simulink model "Copy_of_neural_network_training"  (R2019a)
settings: Solver=FixedStepAuto  StartTime=0.0  StopTime=500  FixedStep=Ts  RelTol=1e-3  EnableMultiTasking=on
values from neighbouring files (symbols this model uses):
  f1_off = 0    [vreflex.m]
  f2_off = 0    [vreflex.m]
  f3_off = 0    [vreflex.m]
  f4_off = 0    [vreflex.m]
  f5_off = 0    [vreflex.m]
  f6_off = 0    [vreflex.m]
  trial = str2double(get(handles.tryno,'String'))    [vreflex.m]
  Ts = 0.0005    [vreflex.m]
  weight = evalin('base','weight')    [vreflex.m]
undefined symbols (not defined in the file or in its folder): filt_den, filt_num, Pull, up
libraries: dspsigops x9, speedgoatlib_IO183 x6, slrtlib x5, dspswit3 x1, dspstat3 x1, simulink x1
settings Model: Creator=vnalam  LastModifiedBy=vnalam
settings DataIOCC: LimitDataPoints=on  SaveFormat=StructureWithTime  ReturnWorkspaceOutputs=off
settings OptimizationCC: BlockReduction=off  OptimizeBlockIOStorage=off  BufferReuse=off  GlobalBufferReuse=off  ExpressionFolding=off  LocalBlockOutputs=off  LifeSpan=inf  OptimizeDataStoreBuffers=off  BusAssignmentInplaceUpdate=off
settings DebuggingCC: AllowSymbolicDim=off  SFUnexpectedBacktrackingDiag=warning  SFNoUnconditionalDefaultTransitionDiag=warning  SFExecutionAtInitializationDiag=none  ArithmeticOperatorsInVariantConditions=warning
settings HardwareCC: ProdBitPerPointer=32  ProdBitPerSizeT=32  ProdBitPerPtrDiffT=32  ProdLargestAtomicFloat=None  ProdWordSize=32  ProdLongLongMode=on  ProdHWDeviceType=Generic->32-bit x86 compatible
settings ModelReferenceCC: PropagateSignalLabelsOutOfModel=off
settings SFSimCC: SimUseLocalCustomCode=off
settings RTWCC: SystemTargetFile=slrt.tlc  TLCOptions=-axPCModelStackSizeKB=512  TemplateMakefile=slrt_default_tmf  Description=Simulink Real-Time  RTWUseLocalCustomCode=off  CodeExecutionProfiling=on  RTWCompilerOptimization=on
settings CodeAppCC: StateflowObjectComments=on
settings SimulinkRealTimeCC: PreserveStateflowLocalDataDimensions=off  xPCisDownloadable=off
settings ConfigComp: CovMetricSettings=dw  CovHtmlReporting=on  CovSaveCumulativeToWorkspaceVar=on  CovSaveSingleToWorkspaceVar=on  CovExternalEMLEnable=off

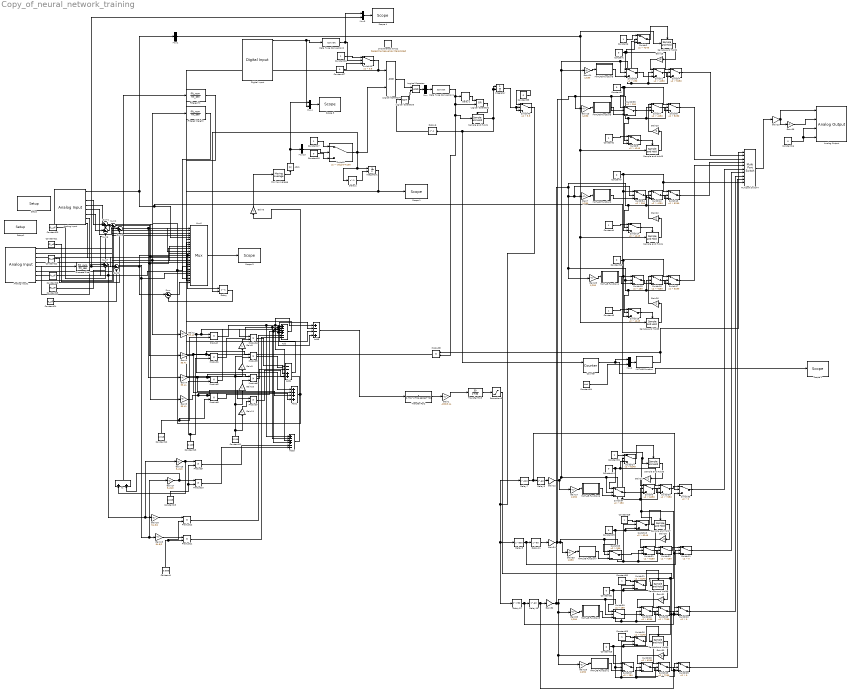
== system Copy_of_neural_network_training ==
  Abs1 : Abs
  Add : Sum  Inputs=+--+--
  Add1 : Sum  Inputs=--++
  Add2 : Sum  Inputs=++++
  Add3 : Sum  Inputs=+--+--
  Add5 : Sum  Inputs=+--+
  Analog Input : speedgoatlib_IO183/Analog Input  Priority=0  parModuleId=1  parSampTime=Ts  parPciSlot=-1  parAdChannelLow=1  parAdChannelHigh=8
      settings: SourceProductName=Simulink Real-Time: Speedgoat Library
  Analog Input1 : speedgoatlib_IO183/Analog Input  Priority=0  parModuleId=2  parSampTime=Ts  parPciSlot=-1  parAdChannelLow=1  parAdChannelHigh=8
      settings: SourceProductName=Simulink Real-Time: Speedgoat Library
  Analog Output : speedgoatlib_IO183/Analog Output  parModuleId=1  parSampTime=-1  parDaSimult=on  parPciSlot=-1  parDaChannels=[1 2 3 4]  parDaInit=[0 0 0 0]  parDaReset=[0 0 0 0]
      settings: SourceProductName=Simulink Real-Time: Speedgoat Library
  Constant{,3,7,10,14..16,18,27,29,31,35} (12 alike) : Constant  Value=0  SampleTime=Ts
  Constant1 : Constant  Value=0.095  SampleTime=-1
  Constant11 : Constant  Value=0.110  SampleTime=-1
  Constant12 : Constant  Value=0.315  SampleTime=-1
  Constant13 : Constant  Value=0.105  SampleTime=-1
  Constant{2,4..6,17,26,28,30,32..33} (10 alike) : Constant  SampleTime=Ts
  Constant19 : Constant  Value=0.025  SampleTime=-1
  Constant20 : Constant  Value=f1_off  SampleTime=Ts
  Constant21 : Constant  Value=f2_off  SampleTime=Ts
  Constant22 : Constant  Value=f3_off  SampleTime=Ts
  Constant23 : Constant  Value=f4_off  SampleTime=Ts
  Constant24 : Constant  Value=f6_off  SampleTime=Ts
  Constant25 : Constant  Value=f5_off  SampleTime=Ts
  Constant34 : Constant  Value=trial  SampleTime=Ts
  Counter : dspswit3/Counter  Direction=Up  CountEvent=Rising edge  CounterSize=User defined  MaxCount=255  InitialCount=0  Output=Count and Hit  HitValue=32  ResetInput=on  SamplesPerFrame=1  Ts=1  CntDtype=double  HitDtype=Boolean
  Data Type Conversion1 : DataTypeConversion
  Data Type Conversion2 : DataTypeConversion
  Delay : Delay  DelayLength=1  ShowEnablePort=on
      settings: InputPortMap=u0,e6
  Delay1 : Delay  DelayLength=12000  InitialCondition=0  SampleTime=Ts
  Delay11 : Delay  DelayLength=60  InitialCondition=0  SampleTime=Ts
  Delay12 : Delay  DelayLength=780  InitialCondition=0  SampleTime=Ts
  Delay13 : Delay  DelayLength=60  InitialCondition=0  SampleTime=Ts
  Delay2 : Delay  DelayLength=1  InitialCondition=0  SampleTime=Ts
  Delay6 : Delay  DelayLength=1  InitialCondition=0  SampleTime=Ts
  Delay7 : Delay  DelayLength=220  InitialCondition=0  SampleTime=Ts
  Delay8 : Delay  DelayLength=500  InitialCondition=0  SampleTime=Ts
  Delay9 : Delay  DelayLength=60  InitialCondition=0  SampleTime=Ts
  Digital Input : speedgoatlib_IO183/Digital Input  parModuleId=2  parSampTime=-1  parPciSlot=-1  parDiChannels=[9 10 11 12 13 14 15 16]
      settings: SourceProductName=Simulink Real-Time: Speedgoat Library
  Discrete Filter : DiscreteFilter  Numerator=filt_num  Denominator=filt_den
  FIltered Fy : DiscreteFilter  Numerator=filt_num  Denominator=filt_den  InputProcessing=Columns as channels (frame based)  FilterStructure=Direct form II transposed  a0EqualsOne=on
  Filtered Weight : DiscreteFilter  Numerator=filt_num  Denominator=filt_den  InputProcessing=Columns as channels (frame based)  FilterStructure=Direct form II transposed  a0EqualsOne=on
  Fy : Sum
  Gain1 : Gain  Gain=-180/3.14
  Gain{8..11} (4 alike) : Gain
  Gain12 : Gain  Gain=2000
  Gain{7,13,24..25,27,29,33,35} (8 alike) : Gain  Gain=1/250
  Gain{15,20..22,26,28,30..31} (8 alike) : Gain  Gain=-2
  Gain{16..19} (4 alike) : Gain  Gain=54.8/2
  Gain{2..5} (4 alike) : Gain  Gain=53.41
  Gain23 : Gain  Gain=1/40
  Gain32 : Gain  Gain=2000
  Gain34 : Gain  Gain=2000
  Gain36 : Gain  Gain=-1
  Gain6 : Gain  Gain=-1
  Integrator : Integrator  ExternalReset=rising
  Integrator1 : Integrator  ExternalReset=falling
  Logical Operator : Logic  AllPortsSameDT=off  OutDataTypeStr=boolean
  Logical Operator2 : Logic  Operator=OR  AllPortsSameDT=off  OutDataTypeStr=boolean
  Logical Operator3 : Logic  Operator=NOT  AllPortsSameDT=off  OutDataTypeStr=boolean
  Logical Operator4 : Logic  AllPortsSameDT=off  OutDataTypeStr=boolean
  MATLAB Function : MATLAB Function  TreatAsAtomicUnit=on
  MATLAB Function1 : MATLAB Function  TreatAsAtomicUnit=on
  MATLAB Function2 : MATLAB Function  TreatAsAtomicUnit=on
  MATLAB Function3 : MATLAB Function  TreatAsAtomicUnit=on
  MATLAB Function4 : MATLAB Function  TreatAsAtomicUnit=on
  MATLAB Function5 : MATLAB Function  TreatAsAtomicUnit=on
  MATLAB Function6 : MATLAB Function  TreatAsAtomicUnit=on
  MATLAB Function7 : MATLAB Function  TreatAsAtomicUnit=on
  MATLAB Function8 : MATLAB Function  TreatAsAtomicUnit=on
  Moving Average : dspstat3/Moving Average  Method=Sliding window  ForgettingFactorPort=off  SpecifyWindowLength=on  WindowLength=8  ForgettingFactor=0.9  SimulateUsing=Code generation
  Multiport Switch4 : MultiPortSwitch  Inputs=9
  Mux : Mux  Inputs=1
  Mux1 : Mux  Inputs=1
  Mux13 : Mux  Inputs=1
  Mux2 : Mux  Inputs=2
  Mux3 : Mux  Inputs=2
  Mux4 : Mux  Inputs=2
  Mux6 : Mux  Inputs=25
      settings: DisplayOption=signals
  Product{,1..12} (13 alike) : Product
  Sample and Hold{1..9} (9 alike) : dspsigops/Sample and Hold  trig=Rising edge  initCond=0  latchinput=off
  Saturation5 : Saturate  UpperLimit=100  LowerLimit=-100
  Scope 1 : slrtlib/Displays and Logging/Scope   scopeno=2  scopetype=Target  autostart=on  viewmode=Graphical sliding  formatstr='%15.6f'  grid=on  ylimits=[0,0]  nosamples=10000  noprepostsamples=0  interleave=1  triggermode=FreeRun  triggersignal=1  trigsignalfromport=off  triggerlevel=0.0  triggerslope=Either  triggerscope=1  triggersample=0  filename=tot303.dat  mode=Lazy  writesize=512  autorestart=off  dynamicfilemode=off  maxwritefilesize=512*1024^2
  Scope 2 : slrtlib/Displays and Logging/Scope   scopeno=1  scopetype=Target  autostart=on  viewmode=Numerical  formatstr='%15.6f'  grid=on  ylimits=[0,0]  nosamples=100  noprepostsamples=0  interleave=1  triggermode=FreeRun  triggersignal=1  trigsignalfromport=off  triggerlevel=0.0  triggerslope=Either  triggerscope=1  triggersample=0  filename=tot303.dat  mode=Lazy  writesize=512  autorestart=off  dynamicfilemode=off  maxwritefilesize=512*1024^2
  Scope 3 : slrtlib/Displays and Logging/Scope   scopeno=3  scopetype=File  autostart=on  viewmode=Graphical redraw  formatstr='%15.6f'  grid=on  ylimits=[0,0]  nosamples=1000000  noprepostsamples=0  interleave=1  triggermode=FreeRun  triggersignal=1  trigsignalfromport=off  triggerlevel=0.0  triggerslope=Either  triggerscope=1  triggersample=0  filename=APW11.dat  mode=Commit  writesize=1024  autorestart=off  dynamicfilemode=off  maxwritefilesize=512*1024^2
  Scope 4 : slrtlib/Displays and Logging/Scope   scopeno=4  scopetype=Target  autostart=on  viewmode=Graphical sliding  formatstr='%15.6f'  grid=on  ylimits=[0,0]  nosamples=20000  noprepostsamples=0  interleave=1  triggermode=FreeRun  triggersignal=1  trigsignalfromport=off  triggerlevel=0.0  triggerslope=Either  triggerscope=1  triggersample=0  filename=tot303.dat  mode=Lazy  writesize=512  autorestart=off  dynamicfilemode=off  maxwritefilesize=512*1024^2
  Scope 5 : slrtlib/Displays and Logging/Scope   scopeno=5  scopetype=Target  autostart=on  viewmode=Graphical sliding  formatstr='%15.6f'  grid=on  ylimits=[0,0]  nosamples=20000  noprepostsamples=0  interleave=1  triggermode=FreeRun  triggersignal=1  trigsignalfromport=off  triggerlevel=0.0  triggerslope=Either  triggerscope=1  triggersample=0  filename=tot303.dat  mode=Lazy  writesize=512  autorestart=off  dynamicfilemode=off  maxwritefilesize=512*1024^2
  Setup : speedgoatlib_IO183/Setup  parModuleId=1  parPciSlot=-1  parDaSimult=on  parAdCoupling=Single Ended  parAdRange=+-10V  parAdChannelLow=1  parAdChannelHigh=8  parDaChannels=[1:4]  parDaRange=0..5V  parDaInit=[0]  parDaReset=[0]  parDoChannels=[1:8]  parDoInit=[0]  parDoReset=[1]  parDiChannels=[9:16]  parIOPullReferenceFront=Pull-up (3.3V)  parIOPullReferenceRear=Pull-up (3.3V)
      settings: SourceProductName=Simulink Real-Time: Speedgoat Library
  Setup1 : speedgoatlib_IO183/Setup  parModuleId=2  parPciSlot=-1  parDaSimult=on  parAdCoupling=Single Ended  parAdRange=+-10V  parAdChannelLow=1  parAdChannelHigh=8  parDaChannels=[1:4]  parDaRange=0..5V  parDaInit=[0]  parDaReset=[0]  parDoChannels=[1:8]  parDoInit=[0]  parDoReset=[1]  parDiChannels=[9:16]  parIOPullReferenceFront=Pull-up (3.3V)  parIOPullReferenceRear=Pull-up (3.3V)
      settings: SourceProductName=Simulink Real-Time: Speedgoat Library
  Sum{,1..3,6..8} (7 alike) : Sum  Inputs=|+-
  Switch{1,7,12,16} (4 alike) : Switch  Criteria=u2 > Threshold  Threshold=4250
  Switch10 : Switch  Criteria=u2 > Threshold  Threshold=0.5
  Switch{11,20,25,33} (4 alike) : Switch  Criteria=u2 > Threshold
  Switch{4,8,13,17} (4 alike) : Switch  Criteria=u2 > Threshold  Threshold=5250
  Switch{2,9,14,18} (4 alike) : Switch  Criteria=u2 > Threshold  Threshold=4245
  Switch{15,27,34..39} (8 alike) : Switch  Criteria=u2 > Threshold  Threshold=250
  Switch{19,21,24,26} (4 alike) : Switch  Criteria=u2 > Threshold  Threshold=6245
  Switch{6,22,28,31} (4 alike) : Switch  Criteria=u2 > Threshold  Threshold=6250
  Switch{23,29..30,32} (4 alike) : Switch  Criteria=u2 > Threshold  Threshold=7250
  Switch40 : Switch  Criteria=u2 > Threshold  Threshold=5.9
  Switch5 : Switch  Criteria=u2 > Threshold  Threshold=weight*4/100
  Transfer Fcn2 : TransferFcn  Numerator=[1 0]  Denominator=[0.75 36.6606 700]
  Transfer Fcn3 : TransferFcn  Numerator=[30]  Denominator=[1 30]
  smoothened ramp2 : simulink/Sources/Repeating Sequence Interpolated  OutValues="[0 1 1 0  0 ].'"  TimeValues=[0 0.0001 1.001 1.002 6.5].'  LookUpMeth=Interpolation-Use End Values  tsamp=Ts  OutMin=[]  OutMax=[]  OutDataTypeStr=double  OutputDataTypeScalingMode=double  OutDataType=fixdt(0,8)  OutScaling=2^-10
  wires:
  Mux6/1 -> Scope 3/1
  Gain2/1 -> Add2/1, Product4/1, Product/1
  Gain3/1 -> Add2/2, Product5/1, Product1/1
  Gain4/1 -> Add2/3, Product6/1, Product2/1
  Gain5/1 -> Add2/4, Product7/1, Product3/1
  Constant11/1 -> Gain8/1, Gain9/1, Gain10/1, Gain11/1
  Gain8/1 -> Product4/2
  Gain9/1 -> Product5/2
  Gain10/1 -> Product6/2
  Gain11/1 -> Product7/2
  Product/1 -> Add3/1, Add5/1, Add/1
  Product1/1 -> Add3/2, Add5/2, Add/2
  Product2/1 -> Add3/3, Add5/3, Add/3
  Product3/1 -> Add5/4, Add/4, Add3/4
  Product4/1 -> Add1/1
  Product6/1 -> Add1/3
  Product5/1 -> Add1/2
  Product7/1 -> Add1/4
  Constant13/1 -> Product2/2, Product1/2
  Constant12/1 -> Product3/2, Product/2
  Add/1 -> Mux6/7
  Add1/1 -> Mux6/8
  Constant17/1 -> Switch5/1
  Constant18/1 -> Switch5/3
  Mux13/1 -> Switch5/2
  Data Type Conversion2/1 -> Mux3/1, Switch10/2
  Constant26/1 -> Switch10/1
  Sum1/1 -> Mux6/9, Gain2/1
  Sum2/1 -> Mux6/10, Gain3/1
  Sum3/1 -> Mux6/11, Gain4/1
  Sum6/1 -> Gain5/1, Mux6/12
  Gain16/1 -> Product9/1, Fy/1
  Constant1/1 -> Product12/2, Product11/2
  Gain17/1 -> Fy/2, Product10/1
  Gain18/1 -> Product12/1
  Gain19/1 -> Product11/1
  Sum8/1 -> Mux6/21, Gain17/1, Gain19/1
  Analog Input1/2 -> Mux6/2
  Analog Input1/3 -> Mux6/3
  Analog Input1/7 -> Mux6/15
  Analog Input1/8 -> Mux6/16
  Analog Input1/1 -> Mux6/1
  Abs1/1 -> Mux4/1, Mux13/1
  Gain6/1 -> Moving Average/1
  Switch5/1 -> Delay2/1, Integrator1/1, Delay/2, Logical Operator4/2
  Mux/1 -> Data Type Conversion1/1
  Delay1/1 -> Logical Operator2/1
  Logical Operator2/1 -> Sample and Hold1/Trigger
  Sample and Hold1/1 -> Counter/1, Delay6/1, Integrator/1, Integrator/2
  Logical Operator/1 -> Mux/1
  Logical Operator3/1 -> Logical Operator/2
  Delay6/1 -> Logical Operator3/1
  Gain12/1 -> Gain27/1, Switch36/2, Switch4/2, Switch1/2, Switch2/2, Gain24/1, Switch37/2, Switch30/2, Switch6/2, Switch24/2
  Data Type Conversion1/1 -> Product8/2, Sample and Hold1/1, Logical Operator2/2, Delay1/1
  Switch1/1 -> Switch4/3
  Gain34/1 -> Gain13/1, Switch35/2, Switch9/2, Switch8/2, Switch7/2, Gain33/1, Switch38/2, Switch31/2, Switch32/2, Switch19/2
  Constant3/1 -> Switch35/1, Switch8/1, Switch9/3
  Switch7/1 -> Switch8/3
  Counter/1 -> Mux2/1, Scope 2/1
  MATLAB Function/1(y) -> Multiport Switch4/1, Product8/1
  Product8/1 -> Mux6/17
  Gain23/1 -> Gain36/1, Analog Output/1
  Constant/1 -> Switch36/1, Switch2/3, Switch4/1
  Constant6/1 -> Switch2/1
  Switch2/1 -> Sample and Hold2/Trigger
  Sample and Hold2/1 -> Gain15/1
  Gain15/1 -> Switch1/1
  Switch9/1 -> Sample and Hold3/Trigger
  Constant2/1 -> Switch9/1
  Sample and Hold3/1 -> Gain20/1
  Gain20/1 -> Switch7/1
  Add2/1 -> Gain6/1, Filtered Weight/1, Mux6/18
  Constant16/1 -> Analog Output/3, Analog Output/4
  Constant7/1 -> Switch34/1, Switch14/3, Multiport Switch4/10, Switch13/1
  Switch12/1 -> Switch13/3
  Switch14/1 -> Sample and Hold4/Trigger
  Constant4/1 -> Switch14/1
  Sample and Hold4/1 -> Gain22/1
  Gain22/1 -> Switch12/1
  Gain25/1 -> MATLAB Function4/1(u)
  Constant10/1 -> Switch17/1, Switch18/3, Switch15/1
  Switch16/1 -> Switch17/3
  Switch15/1 -> Switch16/3
  Switch18/1 -> Sample and Hold5/Trigger
  Constant5/1 -> Switch18/1
  Sample and Hold5/1 -> Gain26/1
  Gain26/1 -> Switch16/1
  MATLAB Function4/1(y) -> Switch15/3
  Mux1/1 -> Sample and Hold5/1, Sample and Hold4/1, Sample and Hold3/1, Sample and Hold2/1
  Analog Input1/4 -> Mux6/4
  Constant27/1 -> Switch10/3
  Switch10/1 -> Logical Operator4/1, Mux6/6
  Constant19/1 -> Product9/2, Product10/2
  Product9/1 -> Add3/5
  Product10/1 -> Add3/6
  Add3/1 -> Mux6/19
  Analog Input/3 -> Sum1/1
  Analog Input/4 -> Sum2/1
  Analog Input/5 -> Sum3/1
  Analog Input/6 -> Sum6/1
  Constant20/1 -> Sum1/2
  Constant21/1 -> Sum2/2
  Constant22/1 -> Sum3/2
  Constant23/1 -> Sum6/2
  Analog Input/7 -> Sum7/1
  Constant25/1 -> Sum7/2
  Analog Input/8 -> Sum8/1
  Constant24/1 -> Sum8/2
  Logical Operator4/1 -> Logical Operator/1
  Switch4/1 -> Multiport Switch4/2
  Switch8/1 -> Multiport Switch4/3
  Switch13/1 -> Multiport Switch4/4
  Switch17/1 -> Multiport Switch4/5
  Multiport Switch4/1 -> Gain23/1
  Gain1/1 -> Transfer Fcn3/1
  Transfer Fcn3/1 -> Saturation5/1
  Delay7/1 -> Delay9/1, Switch33/2
  Constant14/1 -> Switch37/1, Switch24/3, Switch30/1
  Switch6/1 -> Switch30/3
  Sample and Hold6/1 -> Gain21/1
  Switch31/1 -> Switch32/3
  Gain28/1 -> Switch31/1
  Delay8/1 -> Switch11/2, Delay11/1
  Constant32/1 -> Switch24/1
  Switch24/1 -> Sample and Hold6/Trigger
  Gain21/1 -> Switch6/1
  Delay11/1 -> Gain34/1
  Constant28/1 -> Switch19/1
  Constant29/1 -> Switch38/1, Switch19/3, Switch32/1
  Switch19/1 -> Sample and Hold7/Trigger
  Sample and Hold7/1 -> Gain28/1
  Switch22/1 -> Switch23/3
  Gain31/1 -> Switch22/1
  Delay12/1 -> Switch20/2, Delay13/1
  Constant31/1 -> Switch39/1, Switch21/3, Switch23/1
  Switch21/1 -> Sample and Hold8/Trigger
  Sample and Hold8/1 -> Gain31/1
  Switch32/1 -> Switch11/1
  Switch30/1 -> Switch33/1
  Switch23/1 -> Switch20/1
  Constant30/1 -> Switch21/1
  Switch39/1 -> Switch22/3
  Saturation5/1 -> Switch28/3, Switch25/3, Switch20/3, Switch33/3, Switch11/3
  Switch40/1 -> Delay12/1, Delay8/1, Delay7/1
  Gain32/1 -> Gain35/1, Gain29/1, Switch28/2, Switch29/2, Switch26/2, Switch27/2, Switch39/2, Switch22/2, Switch23/2, Switch21/2, Switch34/2, Gain7/1, Gain25/1, Switch18/2, Switch17/2, Switch16/2, Switch15/2, Switch14/2, Switch13/2, Switch12/2
  Gain29/1 -> MATLAB Function1/1(u)
  Switch28/1 -> Switch29/3
  Gain30/1 -> Switch28/1
  MATLAB Function1/1(y) -> Switch27/3
  Delay13/1 -> Switch25/2, Gain32/1
  Constant15/1 -> Switch26/3, Switch29/1, Switch27/1
  Switch26/1 -> Sample and Hold9/Trigger
  Sample and Hold9/1 -> Gain30/1
  Switch29/1 -> Switch25/1
  Analog Input/1 -> Mux6/5, Sample and Hold8/1, Sample and Hold9/1, Sample and Hold7/1, Sample and Hold6/1, Mux1/1
  Constant33/1 -> Switch26/1
  Switch33/1 -> Multiport Switch4/6
  Switch11/1 -> Multiport Switch4/7
  Switch20/1 -> Multiport Switch4/8
  Switch25/1 -> Multiport Switch4/9
  Mux2/1 -> MATLAB Function/1(u)
  Constant34/1 -> Mux2/2
  Delay9/1 -> Gain12/1
  Gain7/1 -> MATLAB Function2/1(u)
  MATLAB Function2/1(y) -> Switch34/3
  Switch34/1 -> Switch12/3
  Gain13/1 -> MATLAB Function3/1(u)
  MATLAB Function3/1(y) -> Switch35/3
  Switch35/1 -> Switch7/3
  Gain24/1 -> MATLAB Function5/1(u)
  MATLAB Function5/1(y) -> Switch36/3
  Switch36/1 -> Switch1/3
  Gain27/1 -> MATLAB Function6/1(u)
  MATLAB Function6/1(y) -> Switch37/3
  Switch37/1 -> Switch6/3
  Gain33/1 -> MATLAB Function7/1(u)
  MATLAB Function7/1(y) -> Switch38/3
  Switch38/1 -> Switch31/3
  Gain35/1 -> MATLAB Function8/1(u)
  MATLAB Function8/1(y) -> Switch39/3
  Integrator/1 -> Switch40/3, Switch40/2
  Constant35/1 -> Switch40/1
  Sum7/1 -> Mux6/20, Gain16/1, Gain18/1
  Gain36/1 -> Analog Output/2
  Analog Input1/6 -> Mux6/14
  Mux4/1 -> Scope 5/1
  Digital Input/1 -> Mux4/2, Data Type Conversion2/1
  Moving Average/1 -> Abs1/1
  Mux3/1 -> Scope 4/1
  Integrator1/1 -> Mux6/22, Scope 1/1
  Delay2/1 -> Integrator1/2
  Transfer Fcn2/1 -> Gain1/1
  Product12/1 -> Add/5
  Product11/1 -> Add/6
  Add5/1 -> Transfer Fcn2/1
  Fy/1 -> FIltered Fy/1
  Filtered Weight/1 -> Mux6/23
  FIltered Fy/1 -> Mux6/24
  Discrete Filter/1 -> Sum/1, Delay/1, Mux6/13, Mux3/2
  Analog Input1/5 -> Discrete Filter/1
  Delay/1 -> Sum/2
  Sum/1 -> Mux6/25

== matlab function Copy_of_neural_network_training/MATLAB Function3 ==
  data: u input; y output
function y = fcn(u)
%#codegen
y=3*((30*u^2-60*u^3+30*u^4))*2000/250;

== matlab function Copy_of_neural_network_training/MATLAB Function5 ==
  data: u input; y output
function y = fcn(u)
%#codegen
y=3*((30*u^2-60*u^3+30*u^4))*2000/250;

== matlab function Copy_of_neural_network_training/MATLAB Function2 ==
  data: u input; y output
function y = fcn(u)
%#codegen
y=3*((30*u^2-60*u^3+30*u^4))*2000/250;

== matlab function Copy_of_neural_network_training/MATLAB Function4 ==
  data: u input; y output
function y = fcn(u)
%#codegen
y=0*((30*u^2-60*u^3+30*u^4))*2000/250;

== matlab function Copy_of_neural_network_training/MATLAB Function ==
  data: u input; y output
function y = fcn(u)
%#codegen
y=0;


if u(1)==1
    y=9;
elseif u(1)==2
    y=8;
elseif u(1)==3
    y=8;
elseif u(1)==4
    y=4;
elseif u(1)==5
    y=4;
elseif u(1)==6
    y=8;
elseif u(1)==7
    y=4;
elseif u(1)==8
    y=8;
elseif u(1)==9
    y=4;
elseif u(1)==10
    y=8;
elseif u(1)==11
    y=8;
elseif u(1)==12
    y=4;
elseif u(1)==13
    y=8;
elseif u(1)==14
    y=4;
elseif u(1)==15
    y=8;
elseif u(1)==16
    y=4;
elseif u(1)==17
    y=8;
elseif u(1)==18
    y=4;
elseif u(1)==19
    y=8;
elseif u(1)==20
    y=4;    
elseif u(1)==21
    y=4;

    
else
    y=0;
end
end

== matlab function Copy_of_neural_network_training/MATLAB Function6 ==
  data: u input; y output
function y = fcn(u)
%#codegen
y=3*((30*u^2-60*u^3+30*u^4))*2000/250;

== matlab function Copy_of_neural_network_training/MATLAB Function7 ==
  data: u input; y output
function y = fcn(u)
%#codegen
y=3*((30*u^2-60*u^3+30*u^4))*2000/250;

== matlab function Copy_of_neural_network_training/MATLAB Function8 ==
  data: u input; y output
function y = fcn(u)
%#codegen
y=3*((30*u^2-60*u^3+30*u^4))*2000/250;

== matlab function Copy_of_neural_network_training/MATLAB Function1 ==
  data: u input; y output
function y = fcn(u)
%#codegen
y=3*((30*u^2-60*u^3+30*u^4))*2000/250;
